simulink subsystem "TurbulenceDisturbance"  (R2024b)
settings: Solver=VariableStepAuto  StartTime=0.0  StopTime=10.0  RelTol=1e-3
values from neighbouring files (symbols this model uses):
  q = [u * sin(theta / 2); cos(theta / 2)]    [Deterministic_6DoF_reynolds_quat.m]    (also in Deterministic_6DoF_reynolds_quat_alphabeta.m; MPC_optimal_plots_m_file.m = linspace(0, max(simout.time), num_optim))
  r = sym("r", [3;1])    [State5dof.m]    (also in SymbolicState.m = sym("r", [2;1]))
undefined symbols (not defined in the file or in its folder): F, MIL
libraries: aerolibwind2 x1
settings Model: Creator=thatf  LastModifiedBy=thatf

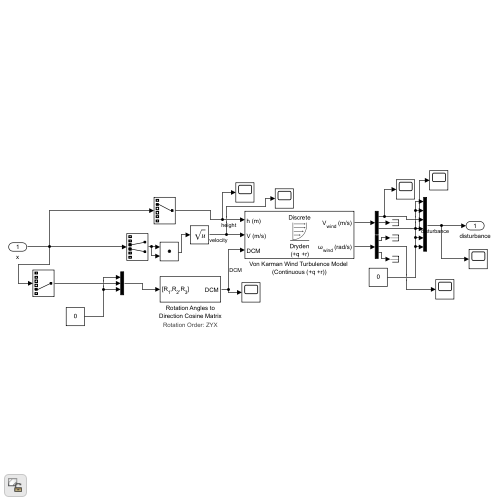
[thumbnail: Simulink's stored preview of the top-level diagram]
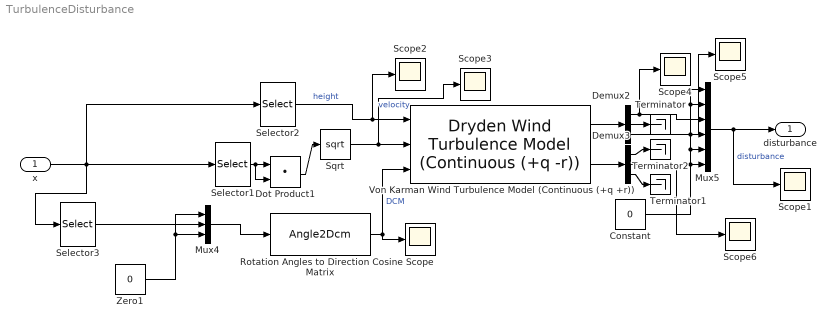
== system TurbulenceDisturbance ==
  x : Inport
  Constant : Constant  Value=0
  Demux2 : Demux  Outputs=3
  Demux3 : Demux  Outputs=3
  Dot Product1 : DotProduct  OutDataTypeStr=Inherit: Inherit via internal rule
  Mux4 : Mux  Inputs=3
  Mux5 : Mux  Inputs=6
  Rotation Angles to Direction Cosine Matrix : Angle2Dcm
      settings: AttributesFormatString=Rotation Order: %<rotationOrder>
  Scope{,1..6} (7 alike) : Scope
  Selector1 : Selector  InputPortWidth=6  IndexOptions=Index vector (dialog)  Indices=[3 4]  OutputSizes=1
  Selector2 : Selector  InputPortWidth=6  IndexOptions=Index vector (dialog)  Indices=[2]  OutputSizes=1
  Selector3 : Selector  InputPortWidth=6  IndexOptions=Index vector (dialog)  Indices=[5]  OutputSizes=1
  Sqrt : Sqrt
  Terminator : Terminator
  Terminator1 : Terminator
  Terminator2 : Terminator
  Von Karman Wind Turbulence Model (Continuous (+q +r)) : aerolibwind2/Dryden Wind Turbulence Model  (Continuous (+q -r))  units=Metric (MKS)  spec=MIL-F-8785C  model=Discrete Dryden (+q +r)  W20=3  Wdeg=0  TurbProb=10^-6  L_high=762  Wingspan=1  ts=0.2  Seed=[23341 23342 23343 23344]  T_on=on
      settings: LibrarySourceBlock=|
      | aerolibwind2/Von Karman Wind Turbulence Model
      | (Continuous (+q +r))
  Zero1 : Constant  Value=0  OutDataTypeStr=Inherit: Inherit via back propagation
  disturbance : Outport
  wires:
  Mux5/1 -> Scope1/1, disturbance/1  "disturbance"
  Selector2/1 -> Von Karman Wind Turbulence Model (Continuous (+q +r))/1, Scope2/1  "height"
  Demux2/3 -> Mux5/4, Scope5/1
  Zero1/1 -> Mux4/1, Mux4/3
  Sqrt/1 -> Von Karman Wind Turbulence Model (Continuous (+q +r))/2, Scope3/1  "velocity"
  Von Karman Wind Turbulence Model (Continuous (+q +r))/1 -> Demux2/1
  Constant/1 -> Mux5/1, Mux5/2, Mux5/5, Mux5/6
  Selector3/1 -> Mux4/2
  Selector1/1 -> Dot Product1/1, Dot Product1/2
  Demux2/1 -> Mux5/3, Scope4/1
  x/1 -> Selector3/1, Selector1/1, Selector2/1
  Rotation Angles to Direction Cosine Matrix/1 -> Scope/1, Von Karman Wind Turbulence Model (Continuous (+q +r))/3  "DCM"
  Demux3/3 -> Terminator1/1
  Mux4/1 -> Rotation Angles to Direction Cosine Matrix/1
  Demux3/1 -> Terminator2/1
  Von Karman Wind Turbulence Model (Continuous (+q +r))/2 -> Demux3/1
  Demux2/2 -> Terminator/1
  Dot Product1/1 -> Sqrt/1
  Demux3/2 -> Scope6/1
